simulink model "RRC_matched"  (R2024a)
settings: Solver=VariableStepDiscrete  StartTime=0.0  StopTime=3200/fs  RelTol=1e-3  EnableMultiTasking=on
PreLoadFcn:
  | %%%%%%%%%%%%%%%%%%%%%%%%%%%%%%%%%%%%%%%%%%%%%%%%%%%%%%%%%%%%%%%%%%%%%%%%%%%
  | % check to see if Simulink library folder is missing from the MATLAB path %
  | %%%%%%%%%%%%%%%%%%%%%%%%%%%%%%%%%%%%%%%%%%%%%%%%%%%%%%%%%%%%%%%%%%%%%%%%%%%
  | if isempty(strfind(path, 'rtlsdr_book_library'))
  | 
  |     % create error window
  |     fig_error = figure(...
  |         'Name', 'Error: RTL-SDR Book Library',...
  |         'Toolbar','none',...
  |         'MenuBar','none',...
  |         'NumberTitle','off',...
  |         'Resize','off',...
  |         'WindowStyle','modal');
  |     fig_error.Position(3) = 600;
  |     fig_error.Position(4) = 150;
  |     fig_axes = axes(...
  |         'Parent',fig_error,...
  |         'Position',[0,0,1,1],...
  |         'visible','off');
  |     % error message
  |     t_title = text(.05,.8,...
  |         'MISSING DIRECTORIES',...
  |         'FontSize',11.5);
  |     t_body = text(.075,.6,...
  |         [{'Simulink cannot find the  \it{<root>}\rm / \it{rtlsdr\_book\_library}\rm  folder in the \it{MATLAB Path}\rm.'},...
  |         {'Please set the MATLAB path following the instructions given in Exercise 2.4.'}],...
  |         'FontSize',10.5);
  |     % buttons
  |     btn_path = uicontrol(...
  |         'Parent',fig_error,...
  |         'String','Set Path Now',...
  |         'FontSize',10,...
  |         'Callback', 'pathtool; close(fig_error);',...
  |         'Position', [fig_error.Position(3)/2-210, 30, 200, 30]);
  |     btn_abort = uicontrol(...
  |         'Parent',fig_error,...
  |         'String','No thanks',...
  |         'FontSize',10,...
  |         'Callback', 'close(fig_error); abort=1;',...
  |         'Position', [fig_error.Position(3)/2+10, 30, 200, 30]);
  | 
  |     % pause to allow user to interact with error box
  |     uiwait(fig_error);
  | 
  |     % abort simulation
  |     try
  |         if abort==1
  |             set_param(gcs, 'SimulationCommand', 'stop');
  |         end
  |     end
  | 
  |     % if user has set path, allow diagram to be updated
  |     if ~exist('abort','var')
  |         % create error window
  |         fig_update = figure(...
  |             'Name', 'Update Diagram',...
  |             'Toolbar','none',...
  |             'MenuBar','none',...
  |             'NumberTitle','off',...
  |             'Resize','off');
  |         fig_update.Position(3) = 400;
  |         fig_update.Position(4) = 120;
  |         fig_axes = axes(...
  |             'Parent',fig_update,...
  |             'Position',[0,0,1,1],...
  |             'visible','off');
  |         % instruction message
  |         t_body = text(.075,.7,...
  |             'Once you have set the path, update the block diagram',...
  |             'FontSize',10.5);
  |         % button
  |         btn_update = uicontrol(...
  |             'Parent',fig_update,...
  |             'String','Update Block Diagram',...
  |             'FontSize',10,...
  |             'Callback', 'set_param(gcs,''SimulationCommand'',''update''); close(gcf)',...
  |             'Position', [fig_update.Position(3)/2-100, 30, 200, 30]);
  |     end
  | 
  |     % clear error components
  |     clear('fig_error','fig_update','fig_axes','t_title','t_body','btn_path','btn_abort','btn_update','abort');
  | 
  | end
  | %%%%%%%%%%%%%%%%%%%%%%%%%%%%%%%%%%%%%%%%%%%%%%%%%%%%%%%%%%%%%%%%%%%%%%%%%%%
  | 
  | MHz = 100;
  | fs = MHz * 1e6;
  | 
  | % parameters for filter design
  | R = 10;               % samples per symbol
  | Symbols = 10;        % symbol periods
  | roll = 0.25;         % rolloff rate
undefined symbols (not defined in the file): fdesignblkfcn, gcbh
libraries: dspsigops x2, commrandsrc3 x1, commdigbbndpm3 x1
CloseFcn:
  | closefcn_model;
Description:
  | Software, Simulation Examples and Design Exercises Licence Agreement
  | 
  | This license agreement refers to the simulation examples, design exercises and files,
  | and associated software MATLAB and Simulink resources that accompany the book:
  | 
  |      Title: Software Defined Radio using MATLAB & Simulink and the RTL-SDR
  |      Published by Strathclyde Academic Media, 2015
  |      Authored by Robert W. Stewart, Kenneth W. Barlee, Dale S.W. Atkinson,
  |      and Louise H. Crockett
  | 
  | and made available as a download from, www.desktopSDR.com or variously acquired
  | by other means such as via USB storage, cloud storage, disk or any other electronic
  | or optical or magnetic storage mechanism. These files and associated software may
  | be used subject to the terms of agreement of the conditions below:
  | 
  |     Copyright © 2015 Robert W. Stewart, Kenneth W. Barlee, Dale S.W. Atkinson,
  |     and Louise H. Crockett
  |     All rights reserved.
  | 
  | Redistribution and use in source and binary forms, with or without modification, are
  | permitted provided that the following conditions are met:
  | 
  |    1.  Redistributions of source code must retain the above copyright notice, this list of
  |         conditions and the following disclaimer.
  | 
  |    2.  Redistributions in binary form must reproduce the above copyright notice, this
  |         list of conditions and the following disclaimer in the documentation and/or other
  |         materials provided with the distribution.
  | 
  |    3.  Neither the name of the copyright holder nor the names of its contributors may
  |         be used to endorse or promote products derived from this software without
  |         specific prior written permission.
  | 
  |    4.  In all cases, the software is, and all modifications and derivatives of the
  |         software shall be, licensed to you solely for use in conjunction with The
  |         MathWorks, Inc. products and service offerings.
  | 
  | THIS SOFTWARE IS PROVIDED BY THE COPYRIGHT HOLDERS AND CONTRIBUTORS
  | "AS IS" AND ANY EXPRESS OR IMPLIED WARRANTIES, INCLUDING, BUT NOT LIMITED
  | TO, THE IMPLIED WARRANTIES OF MERCHANTABILITY AND FITNESS FOR A
  | PARTICULAR PURPOSE ARE DISCLAIMED. IN NO EVENT SHALL THE COPYRIGHT
  | HOLDER OR CONTRIBUTORS BE LIABLE FOR ANY DIRECT, INDIRECT, INCIDENTAL,
  | SPECIAL, EXEMPLARY, OR CONSEQUENTIAL DAMAGES (INCLUDING, BUT NOT
  | LIMITED TO, PROCUREMENT OF SUBSTITUTE GOODS OR SERVICES; LOSS OF USE,
  | DATA, OR PROFITS; OR BUSINESS INTERRUPTION) HOWEVER CAUSED AND ON ANY
  | THEORY OF LIABILITY, WHETHER IN CONTRACT, STRICT LIABILITY, OR TORT
  | (INCLUDING NEGLIGENCE OR OTHERWISE) ARISING IN ANY WAY OUT OF THE USE
  | OF THIS SOFTWARE, EVEN IF ADVISED OF THE POSSIBILITY OF SUCH DAMAGE.
  | 
  | 
  | Audio Tracks used in Simulations Examples and Design Exercises
  | 
  | The music and vocal files used within the Examples files and software within the book
  | were variously written, arranged, performed, recorded and produced by Garrey Rice,
  | Adam Struth, Jamie Struth, Iain Thistlethwaite and also Marshall Craigmyle who
  | collectively, and individually where appropriate, assert and retain all of their copyright,
  | performance and artistic rights. Permission to use and reproduce this music is
  | granted for all purposes associated with MATLAB and Simulink software and the
  | simulation examples and design exercises files that accompany this book. Requests to
  | use the music for any other purpose should be directed to: info@desktopSDR.com.
  | For information on music track names, full credits, and links to the musicians please
  | refer to www.desktopSDR.com/more/audio.
settings Model: Creator=desktopSDR Team  LastModifiedBy=april
settings SolverCC: AlgebraicLoopSolver=TrustRegion
settings DataIOCC: SaveFormat=Array  SaveOutput=off  SignalLogging=off  SaveTime=off  ReturnWorkspaceOutputs=off
settings OptimizationCC: BlockReduction=off  ConditionallyExecuteInputs=off  DefaultParameterBehavior=Inlined  LifeSpan=inf
settings DebuggingCC: AlgebraicLoopMsg=error  UnderspecifiedInitializationDetection=Classic  MergeDetectMultiDrivingBlocksExec=none  SolverPrmCheckMsg=warning  UnconnectedInputMsg=warning  UnconnectedOutputMsg=warning  UnconnectedLineMsg=warning  SFUnexpectedBacktrackingDiag=warning  SFNoUnconditionalDefaultTransitionDiag=warning  SFExecutionAtInitializationDiag=none  ArithmeticOperatorsInVariantConditions=warning
settings HardwareCC: ProdBitPerPointer=32  ProdBitPerSizeT=32  ProdBitPerPtrDiffT=32  ProdLargestAtomicFloat=None  ProdIntDivRoundTo=Undefined  ProdEndianess=Unspecified  ProdWordSize=32  ProdHWDeviceType=ASIC/FPGA->ASIC/FPGA  ProdEqTarget=off
settings ModelReferenceCC: EnableRefExpFcnMdlSchedulingChecks=on  PropagateSignalLabelsOutOfModel=off
settings SFSimCC: SimUseLocalCustomCode=off  CustomCodeUndefinedFunction=UseInterfaceOnly
settings RTWCC: RTWUseLocalCustomCode=off  GPUComputeCapability=3.5  DLArmComputeVersion=19.05
settings CodeAppCC: StateflowObjectComments=on
settings GRTTargetCC: TargetLangStandard=C89/C90 (ANSI)
settings ConfigComp: CovMetricSettings=dw  CovSaveCumulativeToWorkspaceVar=on  CovSaveSingleToWorkspaceVar=on  CovExternalEMLEnable=off  CovSFcnEnable=off

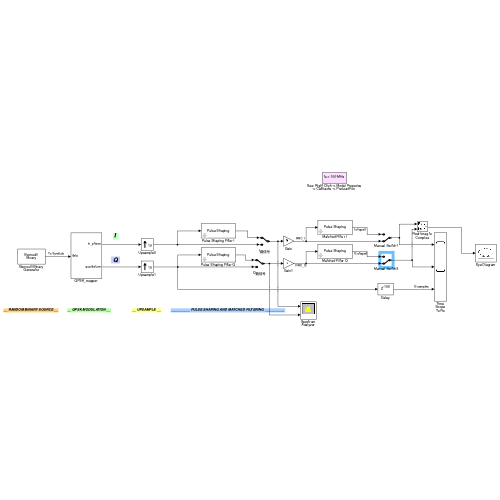
[thumbnail: Simulink's stored preview of the top-level diagram]
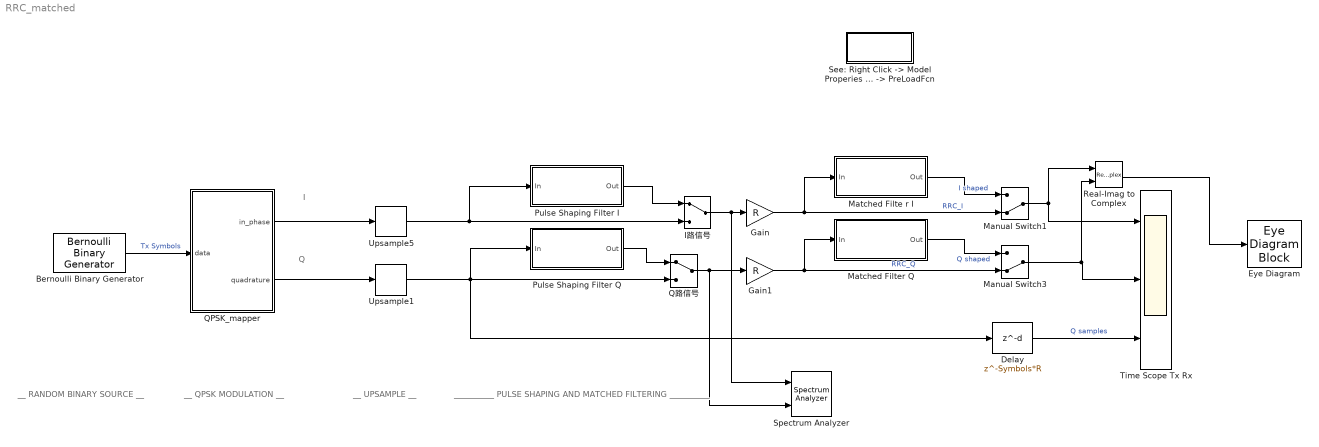
== system RRC_matched ==
  note: I
  note: Q
  note: __ RANDOM BINARY SOURCE __
  note: __ QPSK MODULATION __
  note: __________ PULSE SHAPING AND MATCHED FILTERING __________
  note: __ UPSAMPLE __
  Bernoulli Binary Generator : commrandsrc3/Bernoulli Binary Generator  ProbabilityOfZero=0.5  SeedSource=Auto  Seed=0  SampleTime=(R/2)/fs  SamplesPerFrame=2  OutputDataType=boolean  SimulateUsing=Interpreted execution
  Delay : Delay  DelayLength=Symbols*R  InputProcessing=Columns as channels (frame based)
  Eye Diagram : EyeDiagramBlock  WindowPosition=[516.000000,156.000000,800.000000,500.000000,]  Visible=on  ScopeFrameLocation=window  SamplesPerSymbol=10  YLimits=[-1.5243894304144463,1.5373823346879265]
  Gain : Gain  Gain=R
  Gain1 : Gain  Gain=R
  I路信号 : ManualSwitch
  Manual Switch1 : ManualSwitch  CurrentSetting=0
  Manual Switch3 : ManualSwitch  CurrentSetting=0
  Matched Filte r I : Subsystem  DialogController=fdesignblkfcn  InitFcn=fdesignblkfcn(gcbh, {'InitFcn'});  mask(Pulse Shaping Filter){}
      mask help: Design a Pulse Shaping Filter
      settings: CopyFcn=fdesignblkfcn(gcbh, {'CopyFcn'});
      mask Help: helpview(mapfilelocation('dsp'), 'dsppulseshapingfilter');
      mask Display: disp('Pulse Shaping');
  Matched Filter Q : Subsystem  DialogController=fdesignblkfcn  InitFcn=fdesignblkfcn(gcbh, {'InitFcn'});  mask(Pulse Shaping Filter){}
      mask help: Design a Pulse Shaping Filter
      settings: CopyFcn=fdesignblkfcn(gcbh, {'CopyFcn'});
      mask Help: helpview(mapfilelocation('dsp'), 'dsppulseshapingfilter');
      mask Display: disp('Pulse Shaping');
  Pulse Shaping Filter I : Subsystem  DialogController=fdesignblkfcn  InitFcn=fdesignblkfcn(gcbh, {'InitFcn'});  mask(Pulse Shaping Filter){}
      mask help: Design a Pulse Shaping Filter
      settings: CopyFcn=fdesignblkfcn(gcbh, {'CopyFcn'});
      mask Help: helpview(mapfilelocation('dsp'), 'dsppulseshapingfilter');
      mask Display: disp('Pulse Shaping');
  Pulse Shaping Filter Q : Subsystem  DialogController=fdesignblkfcn  InitFcn=fdesignblkfcn(gcbh, {'InitFcn'});  mask(Pulse Shaping Filter){}
      mask help: Design a Pulse Shaping Filter
      settings: CopyFcn=fdesignblkfcn(gcbh, {'CopyFcn'});
      mask Help: helpview(mapfilelocation('dsp'), 'dsppulseshapingfilter');
      mask Display: disp('Pulse Shaping');
  QPSK_mapper : Subsystem
  Q路信号 : ManualSwitch
  Real-Imag to Complex : RealImagToComplex
  "See: Right Click -> Model Properies -> Callbacks -> PreLoadFcn " : Subsystem
      mask Display:
      | MHz = evalin('base', 'MHz');
      | fprintf(['fs = ',num2str(MHz),' MHz']);
  Spectrum Analyzer : SpectrumAnalyzer  NumInputPorts=2  WindowPosition=[135.000000,208.000000,800.000000,500.000000,]  Visible=on  ScopeFrameLocation=window  YLimits=[-68.48781864,-0.6317109]  ShowLegend=on
  Time Scope Tx Rx : Scope  NumInputPorts=3
  Upsample1 : dspsigops/Upsample  FactorSource=Dialog parameter  N=R  Nmax=16  phase=0  InputProcessing=Columns as channels (frame based)  RateOptions=Allow multirate processing  ic=0  mode=Unused parameter value
  Upsample5 : dspsigops/Upsample  FactorSource=Dialog parameter  N=R  Nmax=16  phase=0  InputProcessing=Columns as channels (frame based)  RateOptions=Allow multirate processing  ic=0  mode=Unused parameter value
  wires:
  Bernoulli Binary Generator/1 -> QPSK_mapper/1(data)  "Tx Symbols"
  QPSK_mapper/2(quadrature) -> Upsample1/1
  Gain/1 -> Manual Switch1/2, Matched Filte r I/1(In)  "RRC_I"
  Gain1/1 -> Manual Switch3/2, Matched Filter Q/1(In)  "RRC_Q"
  QPSK_mapper/1(in_phase) -> Upsample5/1
  Upsample5/1 -> I路信号/2, Pulse Shaping Filter I/1(In)
  Upsample1/1 -> Delay/1, Q路信号/2, Pulse Shaping Filter Q/1(In)
  Delay/1 -> Time Scope Tx Rx/3  "Q samples"
  Pulse Shaping Filter I/1(Out) -> I路信号/1
  I路信号/1 -> Spectrum Analyzer/1, Gain/1
  Matched Filte r I/1(Out) -> Manual Switch1/1  "I shaped"
  Manual Switch1/1 -> Real-Imag to Complex/1, Time Scope Tx Rx/1
  Pulse Shaping Filter Q/1(Out) -> Q路信号/1
  Q路信号/1 -> Spectrum Analyzer/2, Gain1/1
  Matched Filter Q/1(Out) -> Manual Switch3/1  "Q shaped"
  Manual Switch3/1 -> Real-Imag to Complex/2, Time Scope Tx Rx/2
  Real-Imag to Complex/1 -> Eye Diagram/1

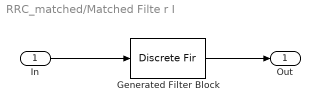
== system RRC_matched/Matched Filte r I ==
  In : Inport
  Generated Filter Block : DiscreteFir  Tag=BlockMethodSubSystem  Coefficients=[-0.00075026359679758816 -0.0010373379379423377 -0.0011580807265444764 -0.0010742686404955528 -0.00077744651516215414 -0.00029330291516455037 0.0003187736524562293 0.00097134174942312514 0.0015594119108653542 0.0019747241194181418 0.0021220659078919381 0.0019354445032959428 0.0013917427084285557 0.00051962253512189652 -0.00059810039808677682 -0.0018296424333794075 -0.003007073952800348 -0.0039458056997003568 -0.0044687578708211334 -0.0044323995319733378 -0.0037513179839879381 -0.002417846461387381 -0.00051359212775869967 0.0017895417631177165 0.0042401191390511262 0.0065296144145032976 0.0083249438340233326 0.0093080846325973906 0.0092186335131371078 0.0078944280166385935 0.0053051647697298409 0.0015743559400942296 -0.0030140415914504848 -0.0080264937649057403 -0.012908572160910946 -0.01702976338459989 -0.019740779307500678 -0.020438104969000427 -0.018629387179611094 -0.013992790859445129 -0.0064237155776998602 0.0039367273182446582 0.016695410593482739 0.031224832169859672 0.046704040587585809 0.062179741050913187 0.076642293869119638 0.089109637467557526 0.098711187556496216 0.10476360210426967 0.10683098861837907 0.10476360210426967 0.098711187556496216 0.089109637467557526 0.076642293869119638 0.062179741050913187 0.046704040587585809 0.031224832169859672 0.016695410593482739 0.0039367273182446582 -0.0064237155776998602 -0.013992790859445129 -0.018629387179611094 -0.020438104969000427 -0.019740779307500678 -0.01702976338459989 -0.012908572160910946 -0.0080264937649057403 -0.0030140415914504848 0.0015743559400942296 0.0053051647697298409 0.0078944280166385935 0.0092186335131371078 0.0093080846325973906 0.0083249438340233326 0.0065296144145032976 0.0042401191390511262 0.0017895417631177165 -0.00051359212775869967 -0.002417846461387381 -0.0037513179839879381 -0.0044323995319733378 -0.0044687578708211334 -0.0039458056997003568 -0.003007073952800348 -0.0018296424333794075 -0.00059810039808677682 0.00051962253512189652 0.0013917427084285557 0.0019354445032959428 0.0021220659078919381 0.0019747241194181418 0.0015594119108653542 0.00097134174942312514 0.0003187736524562293 -0.00029330291516455037 -0.00077744651516215414 -0.0010742686404955528 -0.0011580807265444764 -0.0010373379379423377 -0.00075026359679758816]  InputProcessing=Columns as channels (frame based)
  Out : Outport
  wires:
  Generated Filter Block/1 -> Out/1
  In/1 -> Generated Filter Block/1

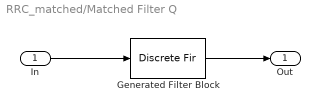
== system RRC_matched/Matched Filter Q ==
  In : Inport
  Generated Filter Block : DiscreteFir  Tag=BlockMethodSubSystem  Coefficients=[-0.00075026359679758816 -0.0010373379379423377 -0.0011580807265444764 -0.0010742686404955528 -0.00077744651516215414 -0.00029330291516455037 0.0003187736524562293 0.00097134174942312514 0.0015594119108653542 0.0019747241194181418 0.0021220659078919381 0.0019354445032959428 0.0013917427084285557 0.00051962253512189652 -0.00059810039808677682 -0.0018296424333794075 -0.003007073952800348 -0.0039458056997003568 -0.0044687578708211334 -0.0044323995319733378 -0.0037513179839879381 -0.002417846461387381 -0.00051359212775869967 0.0017895417631177165 0.0042401191390511262 0.0065296144145032976 0.0083249438340233326 0.0093080846325973906 0.0092186335131371078 0.0078944280166385935 0.0053051647697298409 0.0015743559400942296 -0.0030140415914504848 -0.0080264937649057403 -0.012908572160910946 -0.01702976338459989 -0.019740779307500678 -0.020438104969000427 -0.018629387179611094 -0.013992790859445129 -0.0064237155776998602 0.0039367273182446582 0.016695410593482739 0.031224832169859672 0.046704040587585809 0.062179741050913187 0.076642293869119638 0.089109637467557526 0.098711187556496216 0.10476360210426967 0.10683098861837907 0.10476360210426967 0.098711187556496216 0.089109637467557526 0.076642293869119638 0.062179741050913187 0.046704040587585809 0.031224832169859672 0.016695410593482739 0.0039367273182446582 -0.0064237155776998602 -0.013992790859445129 -0.018629387179611094 -0.020438104969000427 -0.019740779307500678 -0.01702976338459989 -0.012908572160910946 -0.0080264937649057403 -0.0030140415914504848 0.0015743559400942296 0.0053051647697298409 0.0078944280166385935 0.0092186335131371078 0.0093080846325973906 0.0083249438340233326 0.0065296144145032976 0.0042401191390511262 0.0017895417631177165 -0.00051359212775869967 -0.002417846461387381 -0.0037513179839879381 -0.0044323995319733378 -0.0044687578708211334 -0.0039458056997003568 -0.003007073952800348 -0.0018296424333794075 -0.00059810039808677682 0.00051962253512189652 0.0013917427084285557 0.0019354445032959428 0.0021220659078919381 0.0019747241194181418 0.0015594119108653542 0.00097134174942312514 0.0003187736524562293 -0.00029330291516455037 -0.00077744651516215414 -0.0010742686404955528 -0.0011580807265444764 -0.0010373379379423377 -0.00075026359679758816]  InputProcessing=Columns as channels (frame based)
  Out : Outport
  wires:
  In/1 -> Generated Filter Block/1
  Generated Filter Block/1 -> Out/1

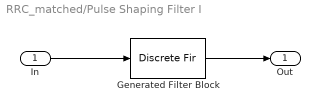
== system RRC_matched/Pulse Shaping Filter I ==
  In : Inport
  Generated Filter Block : DiscreteFir  Tag=BlockMethodSubSystem  Coefficients=[-0.00075026359679758816 -0.0010373379379423377 -0.0011580807265444764 -0.0010742686404955528 -0.00077744651516215414 -0.00029330291516455037 0.0003187736524562293 0.00097134174942312514 0.0015594119108653542 0.0019747241194181418 0.0021220659078919381 0.0019354445032959428 0.0013917427084285557 0.00051962253512189652 -0.00059810039808677682 -0.0018296424333794075 -0.003007073952800348 -0.0039458056997003568 -0.0044687578708211334 -0.0044323995319733378 -0.0037513179839879381 -0.002417846461387381 -0.00051359212775869967 0.0017895417631177165 0.0042401191390511262 0.0065296144145032976 0.0083249438340233326 0.0093080846325973906 0.0092186335131371078 0.0078944280166385935 0.0053051647697298409 0.0015743559400942296 -0.0030140415914504848 -0.0080264937649057403 -0.012908572160910946 -0.01702976338459989 -0.019740779307500678 -0.020438104969000427 -0.018629387179611094 -0.013992790859445129 -0.0064237155776998602 0.0039367273182446582 0.016695410593482739 0.031224832169859672 0.046704040587585809 0.062179741050913187 0.076642293869119638 0.089109637467557526 0.098711187556496216 0.10476360210426967 0.10683098861837907 0.10476360210426967 0.098711187556496216 0.089109637467557526 0.076642293869119638 0.062179741050913187 0.046704040587585809 0.031224832169859672 0.016695410593482739 0.0039367273182446582 -0.0064237155776998602 -0.013992790859445129 -0.018629387179611094 -0.020438104969000427 -0.019740779307500678 -0.01702976338459989 -0.012908572160910946 -0.0080264937649057403 -0.0030140415914504848 0.0015743559400942296 0.0053051647697298409 0.0078944280166385935 0.0092186335131371078 0.0093080846325973906 0.0083249438340233326 0.0065296144145032976 0.0042401191390511262 0.0017895417631177165 -0.00051359212775869967 -0.002417846461387381 -0.0037513179839879381 -0.0044323995319733378 -0.0044687578708211334 -0.0039458056997003568 -0.003007073952800348 -0.0018296424333794075 -0.00059810039808677682 0.00051962253512189652 0.0013917427084285557 0.0019354445032959428 0.0021220659078919381 0.0019747241194181418 0.0015594119108653542 0.00097134174942312514 0.0003187736524562293 -0.00029330291516455037 -0.00077744651516215414 -0.0010742686404955528 -0.0011580807265444764 -0.0010373379379423377 -0.00075026359679758816]  InputProcessing=Columns as channels (frame based)
  Out : Outport
  wires:
  In/1 -> Generated Filter Block/1
  Generated Filter Block/1 -> Out/1

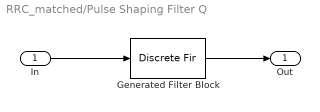
== system RRC_matched/Pulse Shaping Filter Q ==
  In : Inport
  Generated Filter Block : DiscreteFir  Tag=BlockMethodSubSystem  Coefficients=[-0.00075026359679758816 -0.0010373379379423377 -0.0011580807265444764 -0.0010742686404955528 -0.00077744651516215414 -0.00029330291516455037 0.0003187736524562293 0.00097134174942312514 0.0015594119108653542 0.0019747241194181418 0.0021220659078919381 0.0019354445032959428 0.0013917427084285557 0.00051962253512189652 -0.00059810039808677682 -0.0018296424333794075 -0.003007073952800348 -0.0039458056997003568 -0.0044687578708211334 -0.0044323995319733378 -0.0037513179839879381 -0.002417846461387381 -0.00051359212775869967 0.0017895417631177165 0.0042401191390511262 0.0065296144145032976 0.0083249438340233326 0.0093080846325973906 0.0092186335131371078 0.0078944280166385935 0.0053051647697298409 0.0015743559400942296 -0.0030140415914504848 -0.0080264937649057403 -0.012908572160910946 -0.01702976338459989 -0.019740779307500678 -0.020438104969000427 -0.018629387179611094 -0.013992790859445129 -0.0064237155776998602 0.0039367273182446582 0.016695410593482739 0.031224832169859672 0.046704040587585809 0.062179741050913187 0.076642293869119638 0.089109637467557526 0.098711187556496216 0.10476360210426967 0.10683098861837907 0.10476360210426967 0.098711187556496216 0.089109637467557526 0.076642293869119638 0.062179741050913187 0.046704040587585809 0.031224832169859672 0.016695410593482739 0.0039367273182446582 -0.0064237155776998602 -0.013992790859445129 -0.018629387179611094 -0.020438104969000427 -0.019740779307500678 -0.01702976338459989 -0.012908572160910946 -0.0080264937649057403 -0.0030140415914504848 0.0015743559400942296 0.0053051647697298409 0.0078944280166385935 0.0092186335131371078 0.0093080846325973906 0.0083249438340233326 0.0065296144145032976 0.0042401191390511262 0.0017895417631177165 -0.00051359212775869967 -0.002417846461387381 -0.0037513179839879381 -0.0044323995319733378 -0.0044687578708211334 -0.0039458056997003568 -0.003007073952800348 -0.0018296424333794075 -0.00059810039808677682 0.00051962253512189652 0.0013917427084285557 0.0019354445032959428 0.0021220659078919381 0.0019747241194181418 0.0015594119108653542 0.00097134174942312514 0.0003187736524562293 -0.00029330291516455037 -0.00077744651516215414 -0.0010742686404955528 -0.0011580807265444764 -0.0010373379379423377 -0.00075026359679758816]  InputProcessing=Columns as channels (frame based)
  Out : Outport
  wires:
  Generated Filter Block/1 -> Out/1
  In/1 -> Generated Filter Block/1

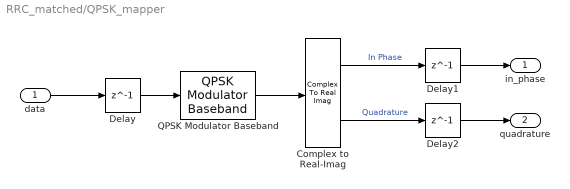
== system RRC_matched/QPSK_mapper ==
  data : Inport
  Complex to Real-Imag : ComplexToRealImag
  Delay : Delay  DelayLength=1  InputProcessing=Columns as channels (frame based)
  Delay1 : Delay  DelayLength=1  InputProcessing=Columns as channels (frame based)
  Delay2 : Delay  DelayLength=1  InputProcessing=Columns as channels (frame based)
  QPSK Modulator Baseband : commdigbbndpm3/QPSK Modulator Baseband  InType=Bit  Enc=Gray  Ph=pi/4  outDtype=double  outWordLen=16  outUDDataType=sfix(16)  outFracLenMode=User-defined  outFracLen=15  outDataTypeStr=double  outLastDataTypeStr=double
  in_phase : Outport
  quadrature : Outport  Port=2
  wires:
  data/1 -> Delay/1
  QPSK Modulator Baseband/1 -> Complex to Real-Imag/1
  Complex to Real-Imag/2 -> Delay2/1  "Quadrature"
  Complex to Real-Imag/1 -> Delay1/1  "In Phase"
  Delay/1 -> QPSK Modulator Baseband/1
  Delay1/1 -> in_phase/1
  Delay2/1 -> quadrature/1

== system RRC_matched/See: Right Click -> Model Properies -> Callbacks -> PreLoadFcn  ==
